simulink model "offGridPowerInverter_Posicast_RepetitiveControl"  (R2022b)
settings: Solver=FixedStepAuto  StartTime=0.0  StopTime=0.3  FixedStep=1e-6  RelTol=1e-3
libraries: spsSeriesRLCBranchLib x10, spsCurrentMeasurementLib x4, spsMosfetLib x4, spsTriangleGeneratorLib x3, spsFourierLib x2, spsRMSLib x2, spsBreakerLib x1, spsDCVoltageSourceLib x1, spsVoltageMeasurementLib x1, spspowerguiLib x1
settings Model: Creator=XIAO  LastModifiedBy=XIAO
settings DataIOCC: ReturnWorkspaceOutputs=off  LoggingToFile=on

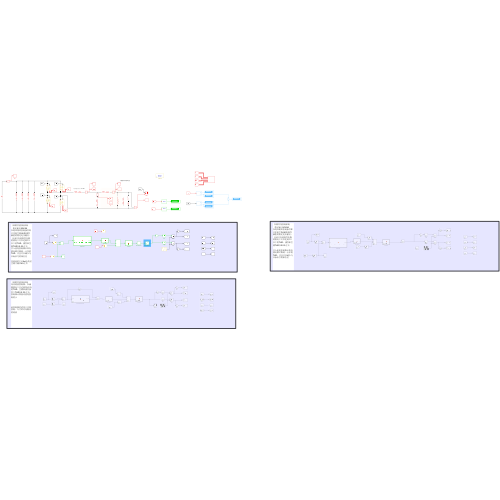
[thumbnail: Simulink's stored preview of the top-level diagram]
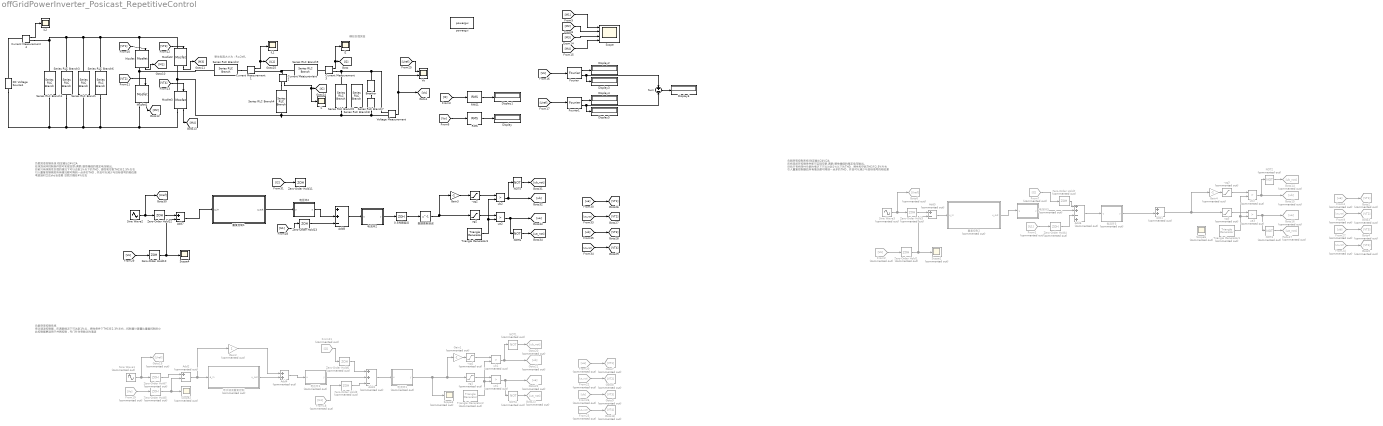
== system offGridPowerInverter_Posicast_RepetitiveControl ==
  note: 寄生电阻大小为：R=2πfL
  note: 模拟负载突变
  note: 负载突变控制系统
      | 奇次谐波控制器，在满载情况下可达到1%以内的THD，空载和感性条件下THD在2.3%左右，控制器计算量比重复控制的小
      |
      | 此控制器更适用于并网控制，专门针对奇数次的谐波
  note: 负载突变控制系统
      | 稳定输出24V/2A
      | 在纯双闭环控制条件即可实现空载/满载/感性幅值的稳定电压输出。
      | 目前只有纯阻性负载的情况下可以达到1％以下的THD，感性和空载THD在2.5%左右
      | 引入重复控制器后所有情况都可降到一点多的THD，并且可以减少与目标信号的相位差
      |
      | 考虑延时之后thd会变差
      | 空载大概在4%左右
  note: 负载突变控制系统
      | 稳定输出24V/2A
      | 在纯双闭环控制条件即可实现空载/满载/感性幅值的稳定电压输出。
      | 目前只有纯阻性负载的情况下可以达到1％以下的THD，感性和空载THD在2.5%左右
      |
      | 引入重复控制器后所有情况都可降到一点多的THD，并且可以减少与目标信号的相位差
  -ug1 : Saturate  Commented=on  UpperLimit=1  LowerLimit=-1
  -ug2 : Saturate  UpperLimit=1  LowerLimit=-1
  -ug3 : Saturate  Commented=on  UpperLimit=1  LowerLimit=-1
  0.5周期延迟 : ZeroOrderHold  SampleTime=5e-5
  Add1 : Sum  Commented=on
  Add2 : Sum  Commented=on  Inputs=+-
  Add3 : Sum  Commented=on  Inputs=++-
  Add4 : Sum  Commented=on
  Add5 : Sum  Commented=on  Inputs=+-
  Add6 : Sum  Commented=on  Inputs=++-+
  Add7 : Sum  Inputs=+-
  Add8 : Sum  Inputs=++-
  Breaker : spsBreakerLib/Breaker  InitialState=0  SwitchingTimes=0.1  External=off  BreakerResistance=0.01  SnubberResistance=1e9  SnubberCapacitance=0  Measurements=None  MoreParameters=on  NoBreakLoop=off
  Current Measurement{1..4} (4 alike) : spsCurrentMeasurementLib/Current Measurement  PhasorSimulation=off  OutputType=Complex  PSBequivalent=0
  DC Voltage Source1 : spsDCVoltageSourceLib/DC Voltage Source  Amplitude=45  Measurements=None
  Display{,1..6} (7 alike) : Display
  Fourier : spsFourierLib/Fourier  Freq=50  n=1  InInit=[0, 0]  Ts=0.0001
  Fourier1 : spsFourierLib/Fourier  Freq=50  n=1  InInit=[0, 0]  Ts=0.0001
  From1 : From  Commented=on  GotoTag=IL1
  From18 : From  Commented=on  GotoTag=IL1
  From19 : From  Commented=on  GotoTag=Vo
  From2 : From  Commented=on  GotoTag=Vo
  From20 : From  Commented=on  GotoTag=ua
  From21 : From  Commented=on  GotoTag=I2
  From22 : From  Commented=on  GotoTag=ua_not
  From23 : From  Commented=on  GotoTag=ub_not
  From24 : From  Commented=on  GotoTag=ub_not
  From26 : From  Commented=on  GotoTag=ub
  From27 : From  Commented=on  GotoTag=ub
  From4 : From  Commented=on  GotoTag=ua
  From7 : From  Commented=on  GotoTag=I2
  From9 : From  Commented=on  GotoTag=ua_not
  Gain1 : Gain  Commented=on  Gain=-1
  Gain2 : Gain  Commented=on
  Gain3 : Gain  Gain=-1
  Gain4 : Gain  Commented=on  Gain=-1
  Goto14 : Goto  Commented=on  GotoTag=ub_not
  Goto15 : Goto  Commented=on  GotoTag=ub
  Goto16 : Goto  Commented=on  GotoTag=ua
  Goto17 : Goto  Commented=on  GotoTag=ua_not
  Goto18 : Goto  Commented=on  GotoTag=VT4
  Goto19 : Goto  Commented=on  GotoTag=Uref
  Goto2 : Goto  Commented=on  GotoTag=VT1
  Goto20 : Goto  Commented=on  GotoTag=ub_not
  Goto21 : Goto  Commented=on  GotoTag=ub
  Goto22 : Goto  Commented=on  GotoTag=ua
  Goto23 : Goto  Commented=on  GotoTag=ua_not
  Goto3 : Goto  Commented=on  GotoTag=VT2
  Goto4 : Goto  Commented=on  GotoTag=VT3
  Goto5 : Goto  Commented=on  GotoTag=VT4
  Goto6 : Goto  Commented=on  GotoTag=Uref
  Goto7 : Goto  Commented=on  GotoTag=VT1
  Goto8 : Goto  Commented=on  GotoTag=VT2
  Goto9 : Goto  Commented=on  GotoTag=VT3
  Mosfet{,1..3} (4 alike) : spsMosfetLib/Mosfet  Ron=0.1  Lon=0  Rd=0.01  Vfd=0  IC=0  Rs=1e5  Cs=inf  Measurements=on
  NOT{1..4} (4 alike) : Logic  Commented=on  Operator=NOT  IconShape=distinctive  AllPortsSameDT=off  OutDataTypeStr=boolean
  NOT5 : Logic  Operator=NOT  IconShape=distinctive  AllPortsSameDT=off  OutDataTypeStr=boolean
  NOT6 : Logic  Operator=NOT  IconShape=distinctive  AllPortsSameDT=off  OutDataTypeStr=boolean
  RMS : spsRMSLib/RMS  TrueRMS=on  Freq=50  RMSInit=24  Ts=5e-5
  RMS1 : spsRMSLib/RMS  TrueRMS=on  Freq=50  RMSInit=24  Ts=5e-5
  Scope : Scope  NumInputPorts=4
  Scope{1..3,6} (4 alike) : Scope  Commented=on
  Scope4 : Scope
  Series RLC Branch{,1,3,6} (4 alike) : spsSeriesRLCBranchLib/Series RLC Branch  LConnTagsString=__new0  RConnTagsString=__new0  BranchType=RC  Resistance=0.01  Inductance=0  SetiL0=off  InitialCurrent=0  Capacitance=470e-6  Setx0=off  InitialVoltage=0  Measurements=None
  Series RLC Branch2 : spsSeriesRLCBranchLib/Series RLC Branch  LConnTagsString=__new0  RConnTagsString=__new0  BranchType=RL  Resistance=0.1  Inductance=0.0015  SetiL0=off  InitialCurrent=0  Capacitance=220e-6  Setx0=off  InitialVoltage=0  Measurements=None
  Series RLC Branch4 : spsSeriesRLCBranchLib/Series RLC Branch  LConnTagsString=__new0  RConnTagsString=__new0  BranchType=RC  Resistance=0.01  Inductance=0  SetiL0=off  InitialCurrent=0  Capacitance=10e-6  Setx0=off  InitialVoltage=0  Measurements=None
  Series RLC Branch5 : spsSeriesRLCBranchLib/Series RLC Branch  LConnTagsString=__new0  RConnTagsString=__new0  BranchType=R  Resistance=1e9  Inductance=0.01  SetiL0=off  InitialCurrent=0  Capacitance=22e-6  Setx0=off  InitialVoltage=0  Measurements=None
  Series RLC Branch7 : spsSeriesRLCBranchLib/Series RLC Branch  LConnTagsString=__new0  RConnTagsString=__new0  BranchType=R  Resistance=12  Inductance=0  SetiL0=off  InitialCurrent=0  Capacitance=22e-6  Setx0=off  InitialVoltage=0  Measurements=None
  Series RLC Branch8 : spsSeriesRLCBranchLib/Series RLC Branch  LConnTagsString=__new0  RConnTagsString=__new0  BranchType=RL  Resistance=12  Inductance=10e-3  SetiL0=off  InitialCurrent=0  Capacitance=220e-6  Setx0=off  InitialVoltage=0  Measurements=None
  Series RLC Branch9 : spsSeriesRLCBranchLib/Series RLC Branch  LConnTagsString=__new0  RConnTagsString=__new0  BranchType=RL  Resistance=0.1  Inductance=0.00012  SetiL0=off  InitialCurrent=0  Capacitance=220e-6  Setx0=off  InitialVoltage=0  Measurements=None
  Sine Wave1 : Sin  Commented=on  Amplitude=24*1.414  Frequency=2*50*pi  SampleTime=0
  Sine Wave2 : Sin  Amplitude=24*1.414  Frequency=2*50*pi  SampleTime=0
  Sine Wave3 : Sin  Commented=on  Amplitude=24*1.414  Frequency=2*50*pi  SampleTime=0
  Sum : Sum  Inputs=+-
  Triangle Generator1 : spsTriangleGeneratorLib/Triangle Generator  Commented=on  Freq=10000  Phase=90  Ts=0
  Triangle Generator2 : spsTriangleGeneratorLib/Triangle Generator  Commented=on  Freq=10000  Phase=90  Ts=0
  Triangle Generator3 : spsTriangleGeneratorLib/Triangle Generator  Freq=10000  Phase=90  Ts=0
  Vo : Scope  NumInputPorts=2
  Voltage Measurement : spsVoltageMeasurementLib/Voltage Measurement  PhasorSimulation=off  OutputType=Complex  PSBequivalent=0
  Zero-Order Hold{1..8} (8 alike) : ZeroOrderHold  Commented=on  SampleTime=1e-4
  Zero-Order Hold10 : ZeroOrderHold  SampleTime=5e-5
  Zero-Order Hold11 : ZeroOrderHold  SampleTime=1e-4
  Zero-Order Hold12 : ZeroOrderHold  SampleTime=5e-5
  Zero-Order Hold13 : ZeroOrderHold  SampleTime=5e-5
  i1 : Scope
  i2 : Scope
  iL1 : Scope
  iL2 : Scope
  powergui : spspowerguiLib/powergui  Priority=1  SimulationMode=Discrete  SampleTime=1e-6  frequency=60  Iterations=50  frequencyindice=0  Pbase=100e6  ErrMax=1e-4  UnitsV=kV  UnitsW=MW  buscounter=0  FunctionMessages=off  echomessages=off  EnableUseOfTLC=off  CurrentSourceSwitches=off  DisableSnubberDevices=off  DisableRonSwitches=off  DisableVfSwitches=off  DisplayEquations=off  AutomaticDiscreteSolvers=off  SolverType=Tustin/Backward Euler (TBE)  Interpol=off  ExternalGateDelay=off  methode=off  Ts=100  x0status=blocks  SPID=on  SwTol=0  HookPort=off  NonlinearTolerance=1e-4  nMaxIteration=100  ContinueOnMaxIteration=off  RestoreLinks=warning  ResistiveCurrentMeasurement=off  Frange=[0:2:500]  Ylog=off  Xlog=on  ShowGrid=off  save=off  variable=ZData  structure=0  ZoomFFT=off  StartTime=0.0  cycles=1  DisplayStyle=1  fundamental=60  FreqAxis=off  MaxFrequency=1000  frequencyindicesteady=1  RmsSteady=1  display=off
  ua1 : RelationalOperator  Commented=on  Operator=>  OutDataTypeStr=boolean  RndMeth=Simplest  InputSameDT=off
  ua2 : RelationalOperator  Operator=>  OutDataTypeStr=boolean  RndMeth=Simplest  InputSameDT=off
  ua3 : RelationalOperator  Commented=on  Operator=>  OutDataTypeStr=boolean  RndMeth=Simplest  InputSameDT=off
  ub1 : RelationalOperator  Commented=on  Operator=>  OutDataTypeStr=boolean  RndMeth=Simplest  InputSameDT=off
  ub2 : RelationalOperator  Operator=>  OutDataTypeStr=boolean  RndMeth=Simplest  InputSameDT=off
  ub3 : RelationalOperator  Commented=on  Operator=>  OutDataTypeStr=boolean  RndMeth=Simplest  InputSameDT=off
  ug1 : Saturate  Commented=on  UpperLimit=1  LowerLimit=-1
  ug2 : Saturate  UpperLimit=1  LowerLimit=-1
  ug3 : Saturate  Commented=on  UpperLimit=1  LowerLimit=-1
  奇次谐波重复控制 : MATLAB Function  Commented=on  TreatAsAtomicUnit=on
  数据更新延迟 : Delay  DelayLength=1  SampleTime=5e-5
  电压环1 : MATLAB Function  Commented=on  TreatAsAtomicUnit=on  SystemSampleTime=0.0001
  电压环2 : MATLAB Function  TreatAsAtomicUnit=on  SystemSampleTime=5e-5
  电压环3 : MATLAB Function  Commented=on  TreatAsAtomicUnit=on  SystemSampleTime=0.0001
  电流环1 : MATLAB Function  Commented=on  TreatAsAtomicUnit=on  SystemSampleTime=0.0001
  电流环2 : MATLAB Function  TreatAsAtomicUnit=on  SystemSampleTime=5e-5
  电流环3 : MATLAB Function  Commented=on  TreatAsAtomicUnit=on  SystemSampleTime=0.0001
  重复控制1 : MATLAB Function  TreatAsAtomicUnit=on
  重复控制2 : MATLAB Function  Commented=on  TreatAsAtomicUnit=on
  wires:
  Voltage Measurement/1 -> [Vo], Vo/2
  [VT1] -> Mosfet/1
  [VT2] -> Mosfet1/1
  [VT3] -> Mosfet2/1
  [VT4] -> Mosfet3/1
  Mosfet/1 -> [M1]
  Mosfet2/1 -> [M3]
  Mosfet1/1 -> [M2]
  Mosfet3/1 -> [M4]
  [M1] -> Scope/1
  [M2] -> Scope/2
  [M3] -> Scope/3
  [M4] -> Scope/4
  RMS/1 -> Display/1
  RMS1/1 -> Display1/1
  [Vo] -> RMS/1
  [I2] -> RMS1/1
  Fourier/1 -> Display2/1
  Fourier/2 -> Display3/1, Sum/1
  Fourier1/1 -> Display4/1
  Fourier1/2 -> Sum/2, Display5/1
  [Vo] -> Fourier/1
  [Uref] -> Fourier1/1
  Sum/1 -> Display6/1
  Current Measurement1/1 -> iL1/1, [IL1]
  Current Measurement3/1 -> i2/1, [I2]
  Zero-Order Hold8/1 -> Add3/3
  From19/1 -> Zero-Order Hold5/1
  Zero-Order Hold6/1 -> Add3/1
  From22/1 -> Goto8/1
  Zero-Order Hold7/1 -> Add2/1
  From18/1 -> Zero-Order Hold8/1
  电压环1/1(y) -> Add3/2
  ua1/1 -> NOT4/1, Goto22/1
  Triangle Generator2/1 -> ua1/2, ub1/2
  ug1/1 -> ua1/1
  NOT1/1 -> Goto20/1
  From20/1 -> Goto7/1
  Add3/1 -> 电流环1/1(u)
  NOT4/1 -> Goto23/1
  -ug1/1 -> ub1/1
  From23/1 -> Goto18/1
  From26/1 -> Goto9/1
  ub1/1 -> NOT1/1, Goto21/1
  From21/1 -> Zero-Order Hold6/1
  Gain1/1 -> -ug1/1
  电流环1/1(y) -> Scope3/1, ug1/1, Gain1/1
  Zero-Order Hold5/1 -> Scope2/1, Add2/2
  Sine Wave1/1 -> Zero-Order Hold7/1, Goto19/1
  Gain2/1 -> Add4/1
  奇次谐波重复控制/1(u_out) -> Add4/2
  Add4/1 -> 电压环1/1(u)
  Add2/1 -> Gain2/1, 奇次谐波重复控制/1(e_in)
  Current Measurement2/1 -> i1/1, [IC]
  [IL1] -> Zero-Order Hold13/1
  Zero-Order Hold10/1 -> Add7/2, Scope4/1
  Add8/1 -> 电流环2/1(u)
  ub2/1 -> NOT5/1, [ub]
  [ub] -> [VT3]
  NOT5/1 -> [ub_not]
  [ua] -> [VT1]
  NOT6/1 -> [ua_not]
  -ug2/1 -> ub2/1
  Sine Wave2/1 -> Zero-Order Hold12/1, [Uref]
  Gain3/1 -> -ug2/1
  ug2/1 -> ua2/1
  Triangle Generator3/1 -> ua2/2, ub2/2
  [I2] -> Zero-Order Hold11/1
  [ub_not] -> [VT4]
  [ua_not] -> [VT2]
  ua2/1 -> NOT6/1, [ua]
  数据更新延迟/1 -> Gain3/1, ug2/1
  电压环2/1(y) -> Add8/2
  [Vo] -> Zero-Order Hold10/1
  Zero-Order Hold13/1 -> Add8/3
  Zero-Order Hold12/1 -> Add7/1
  Zero-Order Hold2/1 -> Add6/1
  Zero-Order Hold4/1 -> Add6/3
  电流环3/1(y) -> Add1/2
  From24/1 -> Goto5/1
  ua3/1 -> NOT3/1, Goto16/1
  Triangle Generator1/1 -> ua3/2, ub3/2
  From9/1 -> Goto3/1
  From7/1 -> Zero-Order Hold2/1
  Sine Wave3/1 -> Zero-Order Hold3/1, Goto6/1
  ug3/1 -> ua3/1
  Gain4/1 -> -ug3/1
  NOT3/1 -> Goto17/1
  From4/1 -> Goto2/1
  -ug3/1 -> ub3/1
  NOT2/1 -> Goto14/1
  From27/1 -> Goto4/1
  ub3/1 -> NOT2/1, Goto15/1
  Add6/1 -> 电流环3/1(u)
  Zero-Order Hold1/1 -> Add5/2, Scope1/1
  Zero-Order Hold3/1 -> Add5/1
  电压环3/1(y) -> Add6/2
  From1/1 -> Zero-Order Hold4/1
  Add5/1 -> 重复控制2/1(u_in)
  重复控制2/1(u_out) -> 电压环3/1(u)
  From2/1 -> Zero-Order Hold1/1
  Add1/1 -> Gain4/1, ug3/1
  电流环2/1(y) -> 0.5周期延迟/1
  Add7/1 -> 重复控制1/1(u_in)
  重复控制1/1(u_out) -> 电压环2/1(u)
  0.5周期延迟/1 -> 数据更新延迟/1
  Current Measurement4/1 -> iL2/1
  [Uref] -> Vo/1
  connections:
  Series RLC Branch1/LConn1 -- Series RLC Branch3/LConn1 -- Series RLC Branch6/LConn1 -- Mosfet2/LConn1 -- Mosfet/LConn1 -- Series RLC Branch/LConn1 -- Current Measurement4/RConn1
  DC Voltage Source1/LConn1 -- Series RLC Branch1/RConn1 -- Series RLC Branch6/RConn1 -- Mosfet3/RConn1 -- Mosfet1/RConn1 -- Series RLC Branch/RConn1 -- Series RLC Branch3/RConn1
  Mosfet/RConn1 -- Mosfet1/LConn1 -- Series RLC Branch2/RConn1
  Mosfet3/LConn1 -- Series RLC Branch7/RConn1 -- Voltage Measurement/LConn2 -- Series RLC Branch5/RConn1 -- Series RLC Branch4/RConn1 -- Mosfet2/RConn1
  Current Measurement1/RConn1 -- Series RLC Branch9/RConn1 -- Current Measurement2/LConn1
  Breaker/LConn1 -- Series RLC Branch7/LConn1
  Series RLC Branch2/LConn1 -- Current Measurement1/LConn1
  Current Measurement3/RConn1 -- Series RLC Branch5/LConn1 -- Breaker/RConn1 -- Voltage Measurement/LConn1
  Current Measurement2/RConn1 -- Series RLC Branch4/LConn1
  Current Measurement4/LConn1 -- DC Voltage Source1/RConn1
  Current Measurement3/LConn1 -- Series RLC Branch9/LConn1

== matlab function offGridPowerInverter_Posicast_RepetitiveControl/电流环3 ==
  settings: updateMethod=DISCRETE
  data: u input; y output
function y = fcn(u)
    % 1. 声明持久变量
    persistent kp ki T y_prev e_prev
    
    % 2. 初始化参数
    kp_init =0.4;     % 比例系数初始值（更合理的范围）
    ki_init = 0;     % 积分系数初始值
    T_init =0.1;   % 10kHz采样对应周期
    
    % 3. 持久变量初始化
    if isempty(kp)
        kp = kp_init;
        ki = ki_init;
        T = T_init;
        y_prev = 0;
        e_prev = 0;
    end
    
    % 4. 正确的离散PI双线性变换公式
    e = u;  % 误差信号
    term1 = y_prev;
    term2 = (kp + ki*T/2) * e;
    term3 = (kp - ki*T/2) * e_prev;
    y = term1 + term2 - term3;
    
    % 5. 更新历史值
    y_prev = y;
    e_prev = e;
end

== matlab function offGridPowerInverter_Posicast_RepetitiveControl/重复控制2 ==
  data: u_in input; u_out output
function u_out = Repetitive_Controller_Internal_Param(u_in)
%REPETITIVE_CONTROLLER_Internal_Param 内部可修改参数的重复控制器
% 功能：
%   可直接在函数内部修改 p、k_rc、N 三个核心参数
%   修复「变量b未完全定义」错误，适配Simulink Coder
% 采样周期：Ts = 1e-4 s（10kHz）

%% ===================== 预定义全局变量（解决未定义错误） =====================
% 提前初始化所有变量，覆盖所有执行路径
persistent x b a;   % 状态变量+系数变量
if isempty(x)
    %% ===================== 1. 在这里修改你的参数 =====================
    N = 200;          % 基波周期采样次数（可改）
    p = 3;            % 相位补偿阶数（可改，例如 p=5）
    k_rc = 0.4;       % 收敛系数（可改，例如 0.3/0.5）
    % ================================================================

    %% ===================== 2. 固定参数 Q(z) = 0.25z + 0.5 + 0.25/z =====================
    Q0 = 0.25;
    Q1 = 0.5;
    Q2 = 0.25;

    %% ===================== 3. 计算延迟阶数 =====================
    delay_order = N - p;  % 分子延迟阶数 = z^(-delay_order)

    %% ===================== 4. 构造分子和分母（显式离散计算） =====================
    max_order = N + 2;    % 统一最大阶数：N+2

    % 强制初始化分子/分母（覆盖所有执行路径）
    b = zeros(1, max_order + 1);  % z降幂：z^0 ~ z^(-max_order)
    a = zeros(1, max_order + 1);
    a(1) = 1.0;  % 分母首项=1

    % 填入分子系数（强制赋值，无分支）
    b(delay_order + 3) = k_rc * Q2;  % z^(-(delay_order+2))
    b(delay_order + 2) = k_rc * Q1;  % z^(-(delay_order+1))
    b(delay_order + 1) = k_rc * Q0;  % z^(-delay_order)

    % 填入分母系数（强制赋值，无分支）
    a(N + 1) = a(N + 1) - Q0;  % z^(-N)
    a(N + 2) = a(N + 2) - Q1;  % z^(-(N+1))
    a(N + 3) = a(N + 3) - Q2;  % z^(-(N+2))

    %% ===================== 5. 初始化状态变量 =====================
    x = zeros(length(a) - 1, 1);
end

%% ===================== 6. 直接II型差分方程（实时计算） =====================
% 输出计算（确保b的长度匹配x）
u_out = b(1) * u_in;
if length(b) > 1
    for i = 2:length(b)
        if i-1 <= length(x)
            u_out = u_out + b(i) * x(i-1);
        end
    end
end

% 状态更新（逐行实现，避免dot函数）
for n = 1:length(x)-1
    x(n) = b(n+1)*u_in - a(n+1)*u_out + x(n+1);
end
x(end) = b(end)*u_in - a(end)*u_out;

end



% % function u_out = Repetitive_Controller_Internal_Param(u_in)
% %REPETITIVE_CONTROLLER_Internal_Param Q=0.9常数版重复控制器
% % 功能：
% %   Q(z)固定为0.9常数（无二阶滤波），仅保留重复控制核心延迟环节
% %   可修改 p、k_rc、N 三个核心参数，适配Simulink Coder
% % 采样周期：Ts = 1e-4 s（10kHz）
% 
% %% ===================== 预定义全局变量（解决未定义错误） =====================
% persistent x b a;   % 状态变量+系数变量
% if isempty(x)
%     %% ===================== 1. 核心参数配置（可修改） =====================
%     N = 200;          % 基波周期采样次数（50Hz基波，10kHz采样→N=200）
%     p = 3;            % 相位补偿阶数
%     k_rc = 0.41;      % 收敛系数
%     Q = 0.9;          % 固定低通常数（替代原二阶Q(z)）
%     % ================================================================
% 
%     %% ===================== 2. 计算延迟阶数 =====================
%     delay_order = N - p;  % 分子延迟阶数 = z^(-delay_order)
% 
%     %% ===================== 3. 构造分子和分母（常数Q版） =====================
%     max_order = N;       % 简化最大阶数（仅保留N阶延迟，无额外滤波阶数）
% 
%     % 强制初始化分子/分母（覆盖所有执行路径）
%     b = zeros(1, max_order + 1);  % z降幂：z^0 ~ z^(-max_order)
%     a = zeros(1, max_order + 1);
%     a(1) = 1.0;  % 分母首项=1
% 
%     % 填入分子系数（仅保留常数Q的延迟项）
%     b(delay_order + 1) = k_rc * Q;  % 分子：k_rc * Q * z^(-delay_order)
% 
%     % 填入分母系数（仅保留常数Q的N阶延迟项）
%     a(N + 1) = a(N + 1) - Q;       % 分母：1 - Q * z^(-N)
% 
%     %% ===================== 4. 初始化状态变量 =====================
%     x = zeros(length(a) - 1, 1);  % 状态变量长度=分母阶数
% end
% 
% %% ===================== 5. 直接II型差分方程（实时计算） =====================
% % 输出计算（确保b的长度匹配x）
% u_out = b(1) * u_in;
% if length(b) > 1
%     for i = 2:length(b)
%         if i-1 <= length(x)
%             u_out = u_out + b(i) * x(i-1);
%         end
%     end
% end
% 
% % 状态更新（逐行实现，避免dot函数，适配代码生成）
% for n = 1:length(x)-1
%     x(n) = b(n+1)*u_in - a(n+1)*u_out + x(n+1);
% end
% x(end) = b(end)*u_in - a(end)*u_out;
% 
% end
%

== matlab function offGridPowerInverter_Posicast_RepetitiveControl/奇次谐波重复控制 ==
  data: u_out output; e_in input
function u_out = ORC_Gm_Fun(e_in)
% ORC_Gm_Fun  实现论文式(12)的离散NORC内模传递函数（Q替换为Q(z)滤波器）
% 输入: e_in   - 误差信号 (标量, Simulink输入)
% 输出: u_out  - 控制量输出 (标量, 给原控制器)
% 固定参数: kr=0.6, m=5, N=200, fs=10kHz (Ts=1e-4)
% 核心修改：Q(z) = 0.25z + 0.5 + 0.25/z (二阶FIR滤波器)

%% 1. 固定参数初始化 (仅首次执行)
persistent kr N m half_N delay_len;
persistent num_S den_S S_len;
persistent Q0 Q1 Q2; % Q(z)滤波器系数
if isempty(kr)
    kr      = 0.6;
    N       = 200;
    m       = 5;
    half_N  = N/2;          % 100
    delay_len = half_N - m; % 95 (对应 z^{-N/2+m} = z^{-95})

%    % Q(z)=0.1705z + 0.6590 + 0.1705/z 系数（截止频率1kHz）
%     Q0 = 0.1705;  % z^1 项系数
%     Q1 = 0.6590;  % z^0 项系数
%     Q2 = 0.1705;  % z^-1 项系数
    
    % Q(z) = 0.25z + 0.5 + 0.25/z 系数   截止频率1.8khz
    Q0 = 0.25;  % z^1 项系数
    Q1 = 0.5;   % z^0 项系数
    Q2 = 0.25;  % z^-1 项系数
    
    % 论文S(z)四阶巴特沃斯低通滤波器系数（长度=5）
    num_S = [0.004824, 0.0193, 0.02895, 0.0193, 0.004824];
    den_S = [1, -2.3695, 2.314, -1.0547, 0.1874];
    S_len = length(num_S);  % 系数总长度=5
end

%% 2. 状态缓存初始化（新增Q(z)滤波缓存）
persistent e_S_buf y_S_buf delay_buf x_iter_buf y_iter_buf;
persistent x_q_buf y_q_buf; % Q(z)输入/输出缓存（长度=2，保存x(n+1)/x(n)/x(n-1)）
if isempty(e_S_buf)
    e_S_buf     = zeros(1, S_len);   % S(z)输入缓存：e(n)~e(n-4)
    y_S_buf     = zeros(1, S_len);   % S(z)输出缓存：y(n)~y(n-4)
    delay_buf   = zeros(1, delay_len);% z^{-95}延迟缓存
    x_iter_buf  = zeros(1, half_N);  % 迭代输入缓存：x(n)~x(n-99)
    y_iter_buf  = zeros(1, half_N);  % 迭代输出缓存：y(n)~y(n-99)
    x_q_buf     = zeros(1, 2);       % Q(z)输入缓存：x(n-1), x(n)
    y_q_buf     = zeros(1, 2);       % Q(z)输出缓存：y(n-1), y(n)
end

%% 3. 步骤1: S(z)低通滤波（逻辑不变）
e_S_buf = [e_in, e_S_buf(1:end-1)]; % 新误差入队
y_S_buf = [0, y_S_buf(1:end-1)];    % 输出缓存移位

% S(z)差分方程
y_S = (sum(num_S .* e_S_buf) - sum(den_S(2:end) .* y_S_buf(2:end))) / den_S(1);
y_S_buf(1) = y_S;

%% 4. 步骤2: 延迟 z^{-N/2 + m} = z^{-95}（逻辑不变）
delay_buf = [y_S, delay_buf(1:end-1)]; % 滤波后信号入队
y_delay = delay_buf(end);             % 延迟95步后的输出

%% 5. 步骤3: 迭代环节 (1-Q(z)z^{-N/2})/(1+Q(z)z^{-N/2})（核心修改）
% 传递函数：(1 + Q(z) z^{-N/2})Y(z) = (1 - Q(z) z^{-N/2})X(z)
% 差分方程：y(n) + Q(z)y(n-N/2) = x(n) - Q(z)x(n-N/2)
% Q(z)x(n) = 0.25x(n+1) + 0.5x(n) + 0.25x(n-1) → 离散域等效为：Q(z)x(n) = 0.25x(n) + 0.5x(n-1) + 0.25x(n-2)

% 1. 更新Q(z)输入缓存（x(n) = y_delay）
x_q_buf = [y_delay, x_q_buf(1)];    % x_q_buf = [x(n), x(n-1)]

% 2. 计算Q(z)滤波后的x(n)和y(n-100)
% Q(z)x(n) = 0.25*x(n) + 0.5*x(n-1) + 0.25*x(n-2)
if length(x_q_buf) < 3
    % 初始化阶段，补0
    Qx_n = Q1 * x_q_buf(1);          % 仅取z^0项
    Qx_n_minus_N2 = Q1 * x_iter_buf(end);
else
    Qx_n = Q0 * x_q_buf(1) + Q1 * x_q_buf(2) + Q2 * x_q_buf(3);
    Qx_n_minus_N2 = Q0 * x_iter_buf(end) + Q1 * x_iter_buf(end-1) + Q2 * x_iter_buf(end-2);
end

% Q(z)y(n-100) = 0.25*y(n-100) + 0.5*y(n-101) + 0.25*y(n-102)
if length(y_iter_buf) < 3
    Qy_n_minus_N2 = Q1 * y_iter_buf(end);
else
    Qy_n_minus_N2 = Q0 * y_iter_buf(end) + Q1 * y_iter_buf(end-1) + Q2 * y_iter_buf(end-2);
end

% 正确计算y(n)
y_iter = y_delay - Qx_n_minus_N2 - Qy_n_minus_N2;

% 2. 更新Q(z)输出缓存
y_q_buf = [y_iter, y_q_buf(1)];

% 3. 更新迭代缓存：新值入队，最老值出队
x_iter_buf = [y_delay, x_iter_buf(1:end-1)];
y_iter_buf = [y_iter, y_iter_buf(1:end-1)];

%% 6. 步骤4: 最终输出（匹配公式负号）
u_out = -kr * y_iter;

end

== matlab function offGridPowerInverter_Posicast_RepetitiveControl/电压环1 ==
  settings: updateMethod=DISCRETE
  data: u input; y output
function y = fcn(u)
    % 1. 声明持久变量
    persistent kp ki T y_prev e_prev
    
    % 2. 初始化参数
    kp_init =0.16;     % 比例系数初始值（更合理的范围）
    ki_init =450;     % 积分系数初始值
    T_init = 0.0001;   % 10kHz采样对应周期
    
    % 3. 持久变量初始化
    if isempty(kp)
        kp = kp_init;
        ki = ki_init;
        T = T_init;
        y_prev = 0;
        e_prev = 0;
    end
    
    % 4. 正确的离散PI双线性变换公式
    e = u;  % 误差信号
    term1 = y_prev;
    term2 = (kp + ki*T/2) * e;
    term3 = (kp - ki*T/2) * e_prev;
    y = term1 + term2 - term3;
    
    % 5. 更新历史值
    y_prev = y;
    e_prev = e;
end

== matlab function offGridPowerInverter_Posicast_RepetitiveControl/电流环1 ==
  settings: updateMethod=DISCRETE
  data: u input; y output
function y = fcn(u)
    % 1. 声明持久变量
    persistent kp ki T y_prev e_prev
    
    % 2. 初始化参数
    kp_init =0.4;     % 比例系数初始值（更合理的范围）
    ki_init = 0;     % 积分系数初始值
    T_init =0.1;   % 10kHz采样对应周期
    
    % 3. 持久变量初始化
    if isempty(kp)
        kp = kp_init;
        ki = ki_init;
        T = T_init;
        y_prev = 0;
        e_prev = 0;
    end
    
    % 4. 正确的离散PI双线性变换公式
    e = u;  % 误差信号
    term1 = y_prev;
    term2 = (kp + ki*T/2) * e;
    term3 = (kp - ki*T/2) * e_prev;
    y = term1 + term2 - term3;
    
    % 5. 更新历史值
    y_prev = y;
    e_prev = e;
end

== matlab function offGridPowerInverter_Posicast_RepetitiveControl/电压环2 ==
  settings: updateMethod=DISCRETE
  data: u input; y output
function y = fcn(u)
    % 1. 声明持久变量
    persistent kp ki T y_prev e_prev
    
    % 2. 初始化参数
    kp_init =0.03;     % 比例系数初始值（更合理的范围）
    ki_init =2800;     % 积分系数初始值
    T_init = 0.0001;   % 10kHz采样对应周期
    
    % 3. 持久变量初始化
    if isempty(kp)
        kp = kp_init;
        ki = ki_init;
        T = T_init;
        y_prev = 0;
        e_prev = 0;
    end
    
    % 4. 正确的离散PI双线性变换公式
    e = u;  % 误差信号
    term1 = y_prev;
    term2 = (kp + ki*T/2) * e;
    term3 = (kp - ki*T/2) * e_prev;
    y = term1 + term2 - term3;
    
    % 5. 更新历史值
    y_prev = y;
    e_prev = e;
end

== matlab function offGridPowerInverter_Posicast_RepetitiveControl/电流环2 ==
  settings: updateMethod=DISCRETE
  data: u input; y output
function y = fcn(u)
    % 1. 声明持久变量
    persistent kp ki T y_prev e_prev
    
    % 2. 初始化参数
    kp_init =0.1;     % 比例系数初始值（更合理的范围）
    ki_init = 0;     % 积分系数初始值
    T_init =0.0001;   % 10kHz采样对应周期
    
    % 3. 持久变量初始化
    if isempty(kp)
        kp = kp_init;
        ki = ki_init;
        T = T_init;
        y_prev = 0;
        e_prev = 0;
    end
    
    % 4. 正确的离散PI双线性变换公式
    e = u;  % 误差信号
    term1 = y_prev;
    term2 = (kp + ki*T/2) * e;
    term3 = (kp - ki*T/2) * e_prev;
    y = term1 + term2 - term3;
    
    % 5. 更新历史值
    y_prev = y;
    e_prev = e;
end

== matlab function offGridPowerInverter_Posicast_RepetitiveControl/重复控制1 ==
  data: u_in input; u_out output
function u_out = Repetitive_Controller_Internal_Param(u_in)
%REPETITIVE_CONTROLLER_Internal_Param 内部可修改参数的重复控制器
% 功能：
%   可直接在函数内部修改 p、k_rc、N 三个核心参数
%   修复「变量b未完全定义」错误，适配Simulink Coder
% 采样周期：Ts = 1e-4 s（10kHz）

%% ===================== 预定义全局变量（解决未定义错误） =====================
% 提前初始化所有变量，覆盖所有执行路径
persistent x b a;   % 状态变量+系数变量
if isempty(x)
    %% ===================== 1. 在这里修改你的参数 =====================
    N = 200;          % 基波周期采样次数（可改）
    p = 3;            % 相位补偿阶数（可改，例如 p=5）
    k_rc = 0.3;       % 收敛系数（可改，例如 0.3/0.5）
    % ================================================================

    %% ===================== 2. 固定参数 Q(z) = 0.25z + 0.5 + 0.25/z =====================
    Q0 = 0.25;
    Q1 = 0.5;
    Q2 = 0.25;

    %% ===================== 3. 计算延迟阶数 =====================
    delay_order = N - p;  % 分子延迟阶数 = z^(-delay_order)

    %% ===================== 4. 构造分子和分母（显式离散计算） =====================
    max_order = N + 2;    % 统一最大阶数：N+2

    % 强制初始化分子/分母（覆盖所有执行路径）
    b = zeros(1, max_order + 1);  % z降幂：z^0 ~ z^(-max_order)
    a = zeros(1, max_order + 1);
    a(1) = 1.0;  % 分母首项=1

    % 填入分子系数（强制赋值，无分支）
    b(delay_order + 3) = k_rc * Q2;  % z^(-(delay_order+2))
    b(delay_order + 2) = k_rc * Q1;  % z^(-(delay_order+1))
    b(delay_order + 1) = k_rc * Q0;  % z^(-delay_order)

    % 填入分母系数（强制赋值，无分支）
    a(N + 1) = a(N + 1) - Q0;  % z^(-N)
    a(N + 2) = a(N + 2) - Q1;  % z^(-(N+1))
    a(N + 3) = a(N + 3) - Q2;  % z^(-(N+2))

    %% ===================== 5. 初始化状态变量 =====================
    x = zeros(length(a) - 1, 1);
end

%% ===================== 6. 直接II型差分方程（实时计算） =====================
% 输出计算（确保b的长度匹配x）
u_out = b(1) * u_in;
if length(b) > 1
    for i = 2:length(b)
        if i-1 <= length(x)
            u_out = u_out + b(i) * x(i-1);
        end
    end
end

% 状态更新（逐行实现，避免dot函数）
for n = 1:length(x)-1
    x(n) = b(n+1)*u_in - a(n+1)*u_out + x(n+1);
end
x(end) = b(end)*u_in - a(end)*u_out;

end



% % function u_out = Repetitive_Controller_Internal_Param(u_in)
% %REPETITIVE_CONTROLLER_Internal_Param Q=0.9常数版重复控制器
% % 功能：
% %   Q(z)固定为0.9常数（无二阶滤波），仅保留重复控制核心延迟环节
% %   可修改 p、k_rc、N 三个核心参数，适配Simulink Coder
% % 采样周期：Ts = 1e-4 s（10kHz）
% 
% %% ===================== 预定义全局变量（解决未定义错误） =====================
% persistent x b a;   % 状态变量+系数变量
% if isempty(x)
%     %% ===================== 1. 核心参数配置（可修改） =====================
%     N = 200;          % 基波周期采样次数（50Hz基波，10kHz采样→N=200）
%     p = 3;            % 相位补偿阶数
%     k_rc = 0.41;      % 收敛系数
%     Q = 0.9;          % 固定低通常数（替代原二阶Q(z)）
%     % ================================================================
% 
%     %% ===================== 2. 计算延迟阶数 =====================
%     delay_order = N - p;  % 分子延迟阶数 = z^(-delay_order)
% 
%     %% ===================== 3. 构造分子和分母（常数Q版） =====================
%     max_order = N;       % 简化最大阶数（仅保留N阶延迟，无额外滤波阶数）
% 
%     % 强制初始化分子/分母（覆盖所有执行路径）
%     b = zeros(1, max_order + 1);  % z降幂：z^0 ~ z^(-max_order)
%     a = zeros(1, max_order + 1);
%     a(1) = 1.0;  % 分母首项=1
% 
%     % 填入分子系数（仅保留常数Q的延迟项）
%     b(delay_order + 1) = k_rc * Q;  % 分子：k_rc * Q * z^(-delay_order)
% 
%     % 填入分母系数（仅保留常数Q的N阶延迟项）
%     a(N + 1) = a(N + 1) - Q;       % 分母：1 - Q * z^(-N)
% 
%     %% ===================== 4. 初始化状态变量 =====================
%     x = zeros(length(a) - 1, 1);  % 状态变量长度=分母阶数
% end
% 
% %% ===================== 5. 直接II型差分方程（实时计算） =====================
% % 输出计算（确保b的长度匹配x）
% u_out = b(1) * u_in;
% if length(b) > 1
%     for i = 2:length(b)
%         if i-1 <= length(x)
%             u_out = u_out + b(i) * x(i-1);
%         end
%     end
% end
% 
% % 状态更新（逐行实现，避免dot函数，适配代码生成）
% for n = 1:length(x)-1
%     x(n) = b(n+1)*u_in - a(n+1)*u_out + x(n+1);
% end
% x(end) = b(end)*u_in - a(end)*u_out;
% 
% end
%

== matlab function offGridPowerInverter_Posicast_RepetitiveControl/电压环3 ==
  settings: updateMethod=DISCRETE
  data: u input; y output
function y = fcn(u)
    % 1. 声明持久变量
    persistent kp ki T y_prev e_prev
    
    % 2. 初始化参数
    kp_init =0.16;     % 比例系数初始值（更合理的范围）
    ki_init =450;     % 积分系数初始值
    T_init = 0.0001;   % 10kHz采样对应周期
    
    % 3. 持久变量初始化
    if isempty(kp)
        kp = kp_init;
        ki = ki_init;
        T = T_init;
        y_prev = 0;
        e_prev = 0;
    end
    
    % 4. 正确的离散PI双线性变换公式
    e = u;  % 误差信号
    term1 = y_prev;
    term2 = (kp + ki*T/2) * e;
    term3 = (kp - ki*T/2) * e_prev;
    y = term1 + term2 - term3;
    
    % 5. 更新历史值
    y_prev = y;
    e_prev = e;
end
